simulink model "Non_Linear_Tank_Tanh"  (R2020a)
settings: Solver=VariableStepAuto  StartTime=0.0  StopTime=sim_time  RelTol=1e-3
undefined symbols (not defined in the file): a_dith, b, c, K, k1, k2, p, w, x1_0, x2_0
settings Model: Creator=jakelangton  LastModifiedBy=jakelangton
settings SolverCC: MaxConsecutiveZCs=100

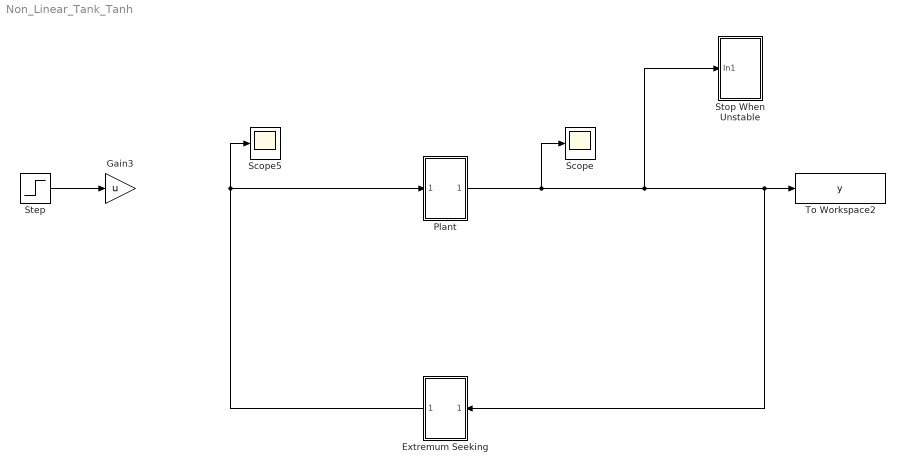
== system Non_Linear_Tank_Tanh ==
  Extremum Seeking : Subsystem
  Gain3 : Gain  Gain=u
  Plant : Subsystem
  Scope : Scope
  Scope5 : Scope
  Step : Step  Before=1  SampleTime=0
  Stop When Unstable : Subsystem
  To Workspace2 : ToWorkspace  VariableName=y  SaveFormat=Timeseries  SampleTime=-1
  wires:
  Step/1 -> Gain3/1
  Extremum Seeking/1(Out1) -> Scope5/1, Plant/1(In1)
  Plant/1(Out1) -> Stop When Unstable/1(In1), Extremum Seeking/1(In1), To Workspace2/1, Scope/1

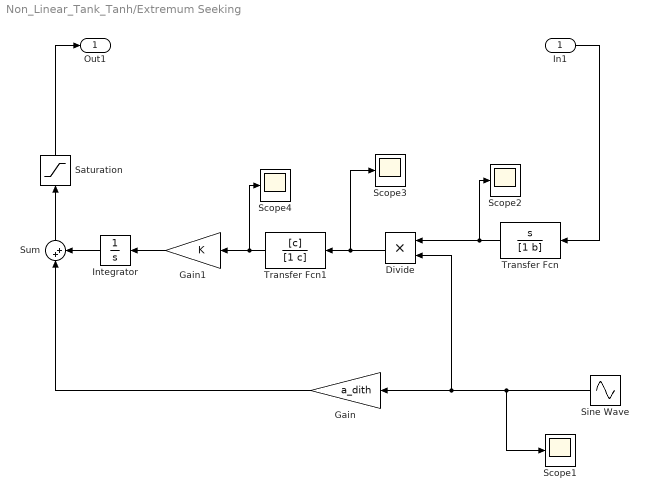
== system Non_Linear_Tank_Tanh/Extremum Seeking ==
  In1 : Inport
  Divide : Product  Inputs=**
  Gain : Gain  Gain=a_dith
  Gain1 : Gain  Gain=K
  Integrator : Integrator
  Saturation : Saturate  UpperLimit=10  LowerLimit=-10
  Scope{1..4} (4 alike) : Scope
  Sine Wave : Sin  Frequency=w  SampleTime=0
  Sum : Sum  Inputs=|++
  Transfer Fcn : TransferFcn  Numerator=[1 0]  Denominator=[1 b]
  Transfer Fcn1 : TransferFcn  Numerator=[c]  Denominator=[1 c]
  Out1 : Outport
  wires:
  In1/1 -> Transfer Fcn/1
  Gain/1 -> Sum/1
  Sum/1 -> Saturation/1
  Saturation/1 -> Out1/1
  Transfer Fcn/1 -> Scope2/1, Divide/1
  Integrator/1 -> Sum/2
  Sine Wave/1 -> Scope1/1, Divide/2, Gain/1
  Gain1/1 -> Integrator/1
  Divide/1 -> Scope3/1, Transfer Fcn1/1
  Transfer Fcn1/1 -> Gain1/1, Scope4/1

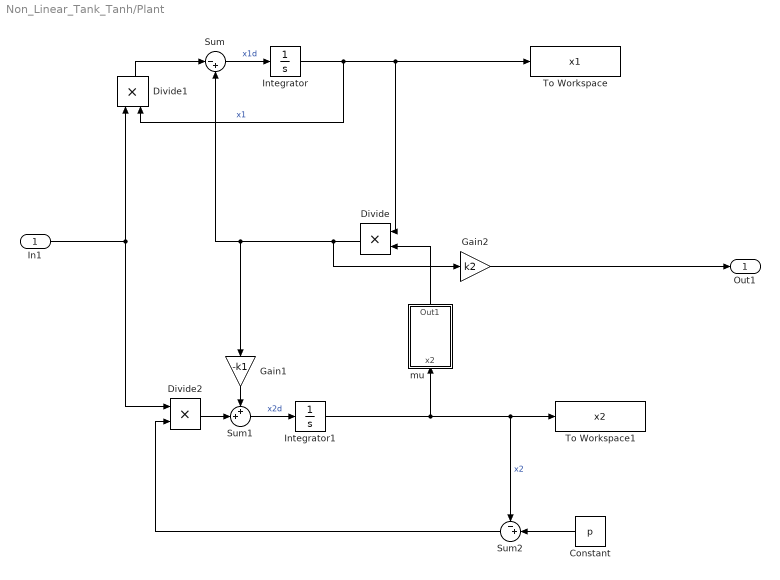
== system Non_Linear_Tank_Tanh/Plant ==
  In1 : Inport
  Constant : Constant  Value=p
  Divide : Product  Inputs=**
  Divide1 : Product  Inputs=**
  Divide2 : Product  Inputs=**
  Gain1 : Gain  Gain=-k1
  Gain2 : Gain  Gain=k2
  Integrator : Integrator  InitialCondition=x1_0
  Integrator1 : Integrator  InitialCondition=x2_0
  Sum : Sum  Inputs=|-+
  Sum1 : Sum  Inputs=++|
  Sum2 : Sum  Inputs=-+|
  To Workspace : ToWorkspace  VariableName=x1  SaveFormat=Timeseries  SampleTime=-1
  To Workspace1 : ToWorkspace  VariableName=x2  SaveFormat=Timeseries  SampleTime=-1
  mu : Subsystem
  Out1 : Outport
  wires:
  Divide2/1 -> Sum1/2
  Sum2/1 -> Divide2/2
  Gain2/1 -> Out1/1
  Sum/1 -> Integrator/1  "x1d"
  Sum1/1 -> Integrator1/1  "x2d"
  In1/1 -> Divide2/1, Divide1/1
  Divide1/1 -> Sum/1
  Gain1/1 -> Sum1/1
  Integrator/1 -> Divide1/2, To Workspace/1, Divide/1  "x1"
  Constant/1 -> Sum2/2
  Divide/1 -> Gain2/1, Sum/2, Gain1/1
  Integrator1/1 -> mu/1(x2), Sum2/1, To Workspace1/1  "x2"
  mu/1(Out1) -> Divide/2

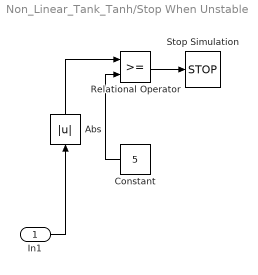
== system Non_Linear_Tank_Tanh/Stop When Unstable ==
  In1 : Inport
  Abs : Abs
  Constant : Constant  Value=5
  Relational Operator : RelationalOperator  OutDataTypeStr=boolean  RndMeth=Simplest
  Stop Simulation : Stop
  wires:
  In1/1 -> Abs/1
  Constant/1 -> Relational Operator/2
  Relational Operator/1 -> Stop Simulation/1
  Abs/1 -> Relational Operator/1

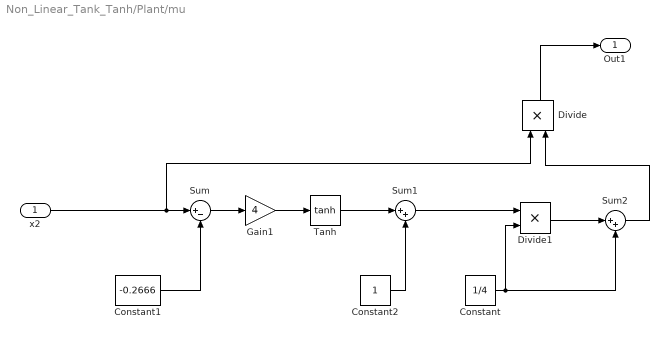
== system Non_Linear_Tank_Tanh/Plant/mu ==
  x2 : Inport
  Constant : Constant  Value=1/4
  Constant1 : Constant  Value=-0.2666
  Constant2 : Constant
  Divide : Product  Inputs=**
  Divide1 : Product  Inputs=**
  Gain1 : Gain  Gain=4
  Sum : Sum  Inputs=|+-
  Sum1 : Sum  Inputs=|++
  Sum2 : Sum  Inputs=|++
  Tanh : Trigonometry  Operator=tanh
  Out1 : Outport
  wires:
  x2/1 -> Divide/1, Sum/1
  Divide/1 -> Out1/1
  Constant1/1 -> Sum/2
  Sum/1 -> Gain1/1
  Gain1/1 -> Tanh/1
  Constant2/1 -> Sum1/2
  Tanh/1 -> Sum1/1
  Sum1/1 -> Divide1/1
  Constant/1 -> Sum2/2, Divide1/2
  Divide1/1 -> Sum2/1
  Sum2/1 -> Divide/2
